simulink model "pr_2_simul"  (R2025b)
settings: Solver=VariableStepAuto  StartTime=0.0  StopTime=60  MaxStep=0.1  RelTol=1e-3
libraries: dspsrcs4 x1
settings Model: Creator=konstantin  LastModifiedBy=konstantin

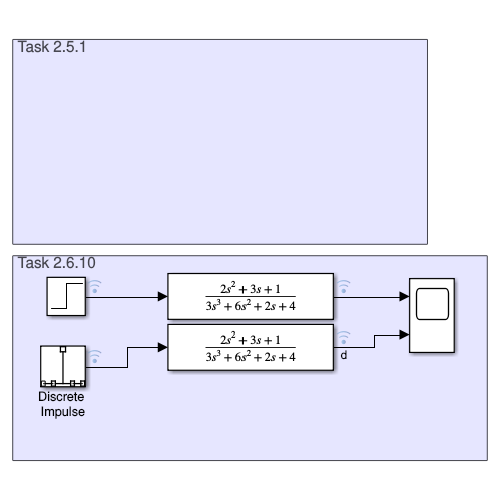
[thumbnail: Simulink's stored preview of the top-level diagram]
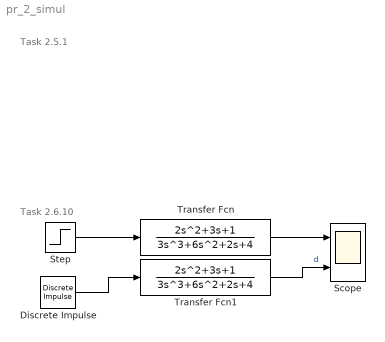
== system pr_2_simul ==
  note: Task 2.5.1
  note: Task 2.6.10
  Discrete Impulse : dspsrcs4/Discrete  Impulse  SFcnStateName=COUNT  Delay=0  SampleTime=1  FrameSample=1  OutputFrames=off  dataType=double  isSigned=on  wordLen=16  udDataType=sfix(16)  fracBitsMode=Best precision  numFracBits=15  OutDataTypeStr=double  LastOutDataTypeStr=double
      settings: SFcnIsStateOwnerBlock=on
  Scope : Scope  NumInputPorts=2
      settings: ActiveDisplayYMinimum=-0.66251953611849279  ActiveDisplayYMaximum=0.88812182790875238
  Step : Step  Time=0  SampleTime=0
  Transfer Fcn : TransferFcn  Numerator=[2 3 1]  Denominator=[3 6 2 4]
  Transfer Fcn1 : TransferFcn  Numerator=[2 3 1]  Denominator=[3 6 2 4]
  wires:
  Step/1 -> Transfer Fcn/1
  Discrete Impulse/1 -> Transfer Fcn1/1
  Transfer Fcn/1 -> Scope/1
  Transfer Fcn1/1 -> Scope/2  "d"
